simulink model "controladorpruebaio3"  (R2025a)
settings: Solver=FixedStepAuto  StartTime=0.0  StopTime=inf  FixedStep=0.015  RelTol=1e-3  EnableMultiTasking=on
libraries: px4Peripheralslib x1, px4uORBlib x1
settings Model: PacingRate=0.790000  ExtModeTrigDuration=10  Creator=The MathWorks, Inc.  LastModifiedBy=aero
settings SolverCC: AlgebraicLoopSolver=TrustRegion  PositivePriorityOrder=on  AutoInsertRateTranBlk=on  MaxZcPerStep=1.0
settings OptimizationCC: EnhancedBackFolding=on  PassReuseOutputArgsAs=Individual arguments  MaxStackSize=64  OptimizeBlockOrder=speed  DifferentSizesBufferReuse=on  OptimizationCustomize=off  EfficientTunableParamExpr=on
settings DebuggingCC: ParameterPrecisionLossMsg=none  ParameterTunabilityLossMsg=error  UnconnectedInputMsg=warning  UnconnectedOutputMsg=warning  UnconnectedLineMsg=warning  SubsystemReferenceDiagnosticForUnitTest=warning  ArithmeticOperatorsInVariantConditions=warning
settings HardwareCC: ProdBitPerPointer=32.0  ProdBitPerSizeT=32.0  ProdBitPerPtrDiffT=32.0  ProdLargestAtomicInteger=Long  ProdLargestAtomicFloat=Double  ProdWordSize=32.0  ProdLongLongMode=on  ProdHWDeviceType=ARM Compatible->ARM Cortex
settings ModelReferenceCC: EnableRefExpFcnMdlSchedulingChecks=on
settings SFSimCC: MATLABDynamicMemAlloc=off  SimTargetLang=C++  SimDLTargetLibrary=mkl-dnn
settings RTWCC: SystemTargetFile=ert.tlc  HardwareBoard=PX4 Pixhawk 6c  TLCOptions="-aInlineSetEventsForThisBaseRateFcn=TLC_FALSE -aSuppressMultiTaskScheduler=TLC_FALSE  -aRateBasedStepFcn=0"  TemplateMakefile=ert_default_tmf  GenerateReport=on  Toolchain=GNU Tools for PX4 Autopilots  IncludeHyperlinkInReport=on  LaunchReport=on  TargetLang=C++  GenerateTraceInfo=on  GenerateTraceReport=on  GenerateTraceReportSl=on  GenerateTraceReportSf=on  GenerateTraceReportEml=on  GPUComputeCapability=3.5  DLArmComputeVersion=19.05  Description=Embedded Coder
settings CodeAppCC: ForceParamTrailComments=on  IgnoreCustomStorageClasses=off  OperatorAnnotations=on  SimulinkDataObjDesc=on  SFDataObjDesc=on  InsertBlockDesc=on
settings ERTTargetCC: ExtModeTransport=3.0  ExtModeStaticAllocSize=1024.0  InlinedParameterPlacement=Hierarchical

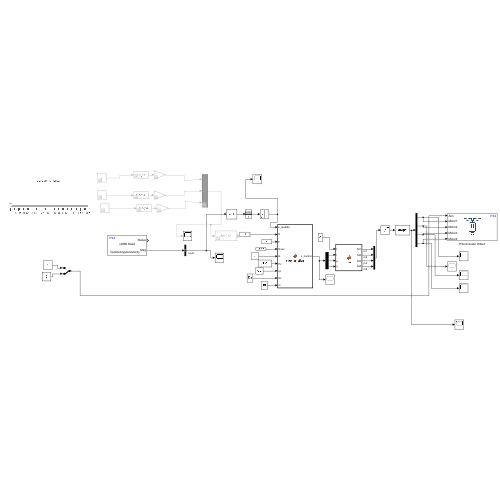
[thumbnail: Simulink's stored preview of the top-level diagram]
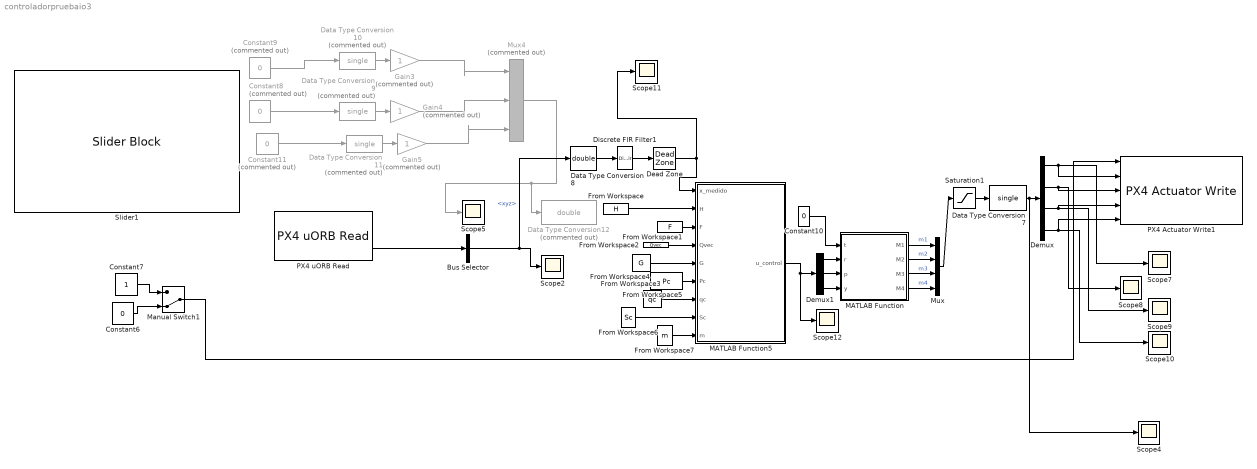
== system controladorpruebaio3 ==
  Bus Selector : BusSelector  OutputSignals=xyz
  Constant10 : Constant  Value=0
  Constant11 : Constant  Commented=on  Value=0
  Constant6 : Constant  Value=0  OutDataTypeStr=boolean
  Constant7 : Constant  OutDataTypeStr=boolean
  Constant8 : Constant  Commented=on  Value=0
  Constant9 : Constant  Commented=on  Value=0
  Data Type Conversion10 : DataTypeConversion  Commented=on  OutDataTypeStr=single  SaturateOnIntegerOverflow=off  RndMeth=Floor
  Data Type Conversion11 : DataTypeConversion  Commented=on  OutDataTypeStr=single  SaturateOnIntegerOverflow=off  RndMeth=Floor
  Data Type Conversion12 : DataTypeConversion  Commented=on  OutDataTypeStr=double  SaturateOnIntegerOverflow=off  RndMeth=Floor  LockScale=on
  Data Type Conversion7 : DataTypeConversion  OutDataTypeStr=single  SaturateOnIntegerOverflow=off  RndMeth=Floor
  Data Type Conversion8 : DataTypeConversion  OutDataTypeStr=double  SaturateOnIntegerOverflow=off  RndMeth=Floor  LockScale=on
  Data Type Conversion9 : DataTypeConversion  Commented=on  OutDataTypeStr=single  SaturateOnIntegerOverflow=off  RndMeth=Floor
  Dead Zone : DeadZone  LowerValue=-0.025  UpperValue=0.025
  Demux : Demux
  Demux1 : Demux  Outputs=3
  Discrete FIR Filter1 : DiscreteFir  Coefficients=[0.2 0.2 0.2 0.2 0.2]
  From Workspace : FromWorkspace  VariableName=H
  From Workspace1 : FromWorkspace  VariableName=F
  From Workspace2 : FromWorkspace  VariableName=Qvec
  From Workspace3 : FromWorkspace  VariableName=qc
  From Workspace4 : FromWorkspace  VariableName=G
  From Workspace5 : FromWorkspace  VariableName=Pc
  From Workspace6 : FromWorkspace  VariableName=Sc
  From Workspace7 : FromWorkspace  VariableName=m
  Gain3 : Gain  Commented=on
  Gain4 : Gain  Commented=on
  Gain5 : Gain  Commented=on
  MATLAB Function : MATLAB Function  TreatAsAtomicUnit=on
  MATLAB Function5 : MATLAB Function  TreatAsAtomicUnit=on
  Manual Switch1 : ManualSwitch  CurrentSetting=0
  Mux : Mux
  Mux4 : Mux  Commented=on  Inputs=3
  PX4 Actuator Write1 : px4Peripheralslib/PX4 Actuator Write  Motor1Enable=on  Motor2Enable=on  Motor3Enable=on  Motor4Enable=on  Motor5Enable=off  Motor6Enable=off  Motor7Enable=off  Motor8Enable=off  Motor9Enable=off  Motor10Enable=off  Motor11Enable=off  Motor12Enable=off  IsMotorArray=off  Servo1Enable=off  Servo2Enable=off  Servo3Enable=off  Servo4Enable=off  Servo5Enable=off  Servo6Enable=off  Servo7Enable=off  Servo8Enable=off  IsServoArray=off
  PX4 uORB Read : px4uORBlib/PX4 uORB Read  uORBTopic=VehicleAngularVelocity  selectInstance=vehicle_angular_velocity  SampleTime=0.015  BlockingMode=off  BlockTimeout=1e-3
  Saturation1 : Saturate  UpperLimit=1  LowerLimit=0
  Scope{2,4..5,7..12} (9 alike) : Scope
      Scope10 settings: ActiveDisplayYMinimum=-0.043109886348247521  ActiveDisplayYMaximum=0.38798897713422775  DataLoggingVariableName=ScopeData10
      Scope11 settings: ActiveDisplayYMinimum=-0.15009255409240721  ActiveDisplayYMaximum=0.01667695045471191  DataLoggingVariableName=ScopeData11
      Scope12 settings: ActiveDisplayYMinimum=-1.0414258708474025  ActiveDisplayYMaximum=1.0153303161323031  DataLoggingVariableName=ScopeData12
      Scope2 settings: ActiveDisplayYMinimum=-0.33577433139146873  ActiveDisplayYMaximum=0.23733546842450437
      Scope4 settings: ActiveDisplayYMinimum=-1.5029836862276127  ActiveDisplayYMaximum=1.9132041073394161  DataLoggingVariableName=ScopeData4
      Scope5 settings: ActiveDisplayYMinimum=-1  ActiveDisplayYMaximum=1  DataLoggingVariableName=ScopeData5
      Scope7 settings: ActiveDisplayYMinimum=0.089401463046669974  ActiveDisplayYMaximum=0.69074354134500027  DataLoggingVariableName=ScopeData7
      Scope8 settings: ActiveDisplayYMinimum=-0.075780542800202952  ActiveDisplayYMaximum=0.76553872250951827  DataLoggingVariableName=ScopeData8
      Scope9 settings: ActiveDisplayYMinimum=0.00290558300912383  ActiveDisplayYMaximum=0.944020101800561  DataLoggingVariableName=ScopeData9
  Slider1 : SliderBlock  ScaleMax=0.6
  wires:
  Demux/4 -> Scope10/1, PX4 Actuator Write1/5
  Data Type Conversion8/1 -> Discrete FIR Filter1/1
  Data Type Conversion7/1 -> Scope4/1, Demux/1
  Constant6/1 -> Manual Switch1/2
  Constant9/1 -> Data Type Conversion10/1
  Gain4/1 -> Mux4/2
  Demux/3 -> Scope9/1, PX4 Actuator Write1/4
  Gain5/1 -> Mux4/3
  Mux4/1 -> Data Type Conversion12/1, Scope5/1
  PX4 uORB Read/2 -> Bus Selector/1
  Gain3/1 -> Mux4/1
  Saturation1/1 -> Data Type Conversion7/1
  Constant7/1 -> Manual Switch1/1
  Data Type Conversion9/1 -> Gain4/1
  Data Type Conversion10/1 -> Gain3/1
  Demux/1 -> Scope7/1, PX4 Actuator Write1/2
  Demux/2 -> Scope8/1, PX4 Actuator Write1/3
  MATLAB Function5/1(u_control) -> Demux1/1, Scope12/1
  Bus Selector/1 -> Scope2/1, Data Type Conversion8/1  "<xyz>"
  Data Type Conversion11/1 -> Gain5/1
  Constant8/1 -> Data Type Conversion9/1
  Constant11/1 -> Data Type Conversion11/1
  Manual Switch1/1 -> PX4 Actuator Write1/1
  Discrete FIR Filter1/1 -> Dead Zone/1
  Dead Zone/1 -> Scope11/1, MATLAB Function5/1(x_medido)
  From Workspace/1 -> MATLAB Function5/2(H)
  From Workspace1/1 -> MATLAB Function5/3(F)
  From Workspace2/1 -> MATLAB Function5/4(Qvec)
  From Workspace4/1 -> MATLAB Function5/5(G)
  From Workspace5/1 -> MATLAB Function5/6(Pc)
  From Workspace3/1 -> MATLAB Function5/7(qc)
  From Workspace6/1 -> MATLAB Function5/8(Sc)
  From Workspace7/1 -> MATLAB Function5/9(m)
  Demux1/1 -> MATLAB Function/2(r)
  Demux1/2 -> MATLAB Function/3(p)
  Demux1/3 -> MATLAB Function/4(y)
  Constant10/1 -> MATLAB Function/1(t)
  MATLAB Function/1(M1) -> Mux/1  "m1"
  MATLAB Function/2(M2) -> Mux/2  "m2"
  MATLAB Function/3(M3) -> Mux/3  "m3"
  MATLAB Function/4(M4) -> Mux/4  "m4"
  Mux/1 -> Saturation1/1

== matlab function controladorpruebaio3/MATLAB Function ==
  data: t input; M1 output; r input; p input; y input; M2 output; M3 output; M4 output
function [M1,M2,M3,M4] = fcn(t, r, p, y)
% t: thrust
% r: roll
% p: pitch
% y: yaw

M1 = t - 0.707107*r - 0.707107*p + y;
M2 = t + 0.707107*r + 0.707107*p + y;
M3 = t + 0.707107*r - 0.707107*p - y;
M4 = t - 0.707107*r + 0.707107*p - y;

== matlab function controladorpruebaio3/MATLAB Function5 ==
  data: x_medido input; u_control output; H input; F input; Qvec input; G input; Pc input; qc input; Sc input; m input
function u_control = mpc_function(x_medido, H, F, Qvec, G, Pc, qc, Sc, m)
    % x_medido: Es el estado que entra desde los sensores/planta en Simulink
    
    % 1. Definir el vector de costo lineal
    f = (2 * x_medido' * F' * Qvec * G)';
    
    % 2. Resolver la optimización para TODO el horizonte
    options = optimoptions('quadprog', 'Display', 'off');
    u_horizonte = quadprog(2*H, f, Pc, qc + Sc * x_medido, [], [], [], [], [], options);
    
    % 3. RETORNAR SOLO LA PRIMERA ACCIÓN (Tamaño m)
    % Si m=1 (una entrada), u_control = u_horizonte(1)
    u_control = u_horizonte(1:m);
end
